simulink model "AD_Stepper_Simulation"  (Simulink 10.0)
settings: Solver=FixedStepDiscrete  StartTime=0.0  StopTime=10  FixedStep=Ts  RelTol=1e-3
InitFcn:
  | Ts = 0.01;      % model sample time
  | Tmax = 0.5;   % maximum time per "tick"
undefined symbols (not defined in the file): AD_Stepper_motor_lib, P_PulsGeber, P_WaveDrive
libraries: simulink x7
settings Model: Creator=Admin  LastModifiedBy=bhisma
settings ConfigSet: Description=rtmc9s12target_R2008a
settings DataIOCC: LimitDataPoints=on  SignalLoggingSaveFormat=ModelDataLogs  SaveOutput=off  SaveTime=off  SignalLoggingName=sigsOut
settings OptimizationCC: ExpressionDepthLimit=2147483647  InitFltsAndDblsToZero=on
settings DebuggingCC: SaveWithParameterizedLinksMsg=none  SignalResolutionControl=TryResolveAllWithWarning  MultiTaskDSMMsg=warning  MultiTaskCondExecSysMsg=none  FcnCallInpInsideContextMsg=warning  StateNameClashWarn=warning
settings HardwareCC: ProdBitPerInt=16  ProdBitPerPointer=16  ProdBitPerSizeT=16  ProdBitPerPtrDiffT=16  ProdEndianess=BigEndian  ProdWordSize=16  ProdHWDeviceType=Motorola HC12  TargetHWDeviceType=32-bit Generic  ProdEqTarget=off
settings RTWCC: GenerateMakefile=off
settings GRTTargetCC: TargetFcnLib=ansi_tfl_tmw.mat  GeneratePreprocessorConditionals=Disable all
settings ConfigComp: CovExternalEMLEnable=off

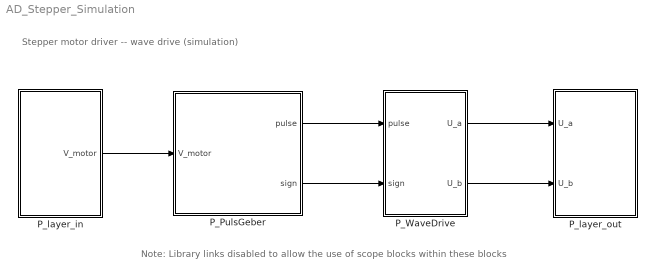
== system AD_Stepper_Simulation ==
  note: Stepper motor driver -- wave drive (simulation)
  note: Note: Library links disabled to allow the use of scope blocks within these blocks
  P_PulsGeber : Subsystem  AncestorBlock=AD_Stepper_motor_lib/P_PulsGeber  TreatAsAtomicUnit=on  SystemSampleTime=Ts
  P_WaveDrive : Subsystem  AncestorBlock=AD_Stepper_motor_lib/P_WaveDrive  TreatAsAtomicUnit=on  SystemSampleTime=Ts
  P_layer_in : Subsystem  TreatAsAtomicUnit=on
  P_layer_out : Subsystem  TreatAsAtomicUnit=on  SystemSampleTime=Ts
  wires:
  P_PulsGeber/1(pulse) -> P_WaveDrive/1(pulse)
  P_PulsGeber/2(sign) -> P_WaveDrive/2(sign)
  P_layer_in/1(V_motor) -> P_PulsGeber/1(V_motor)
  P_WaveDrive/1(U_a) -> P_layer_out/1(U_a)
  P_WaveDrive/2(U_b) -> P_layer_out/2(U_b)

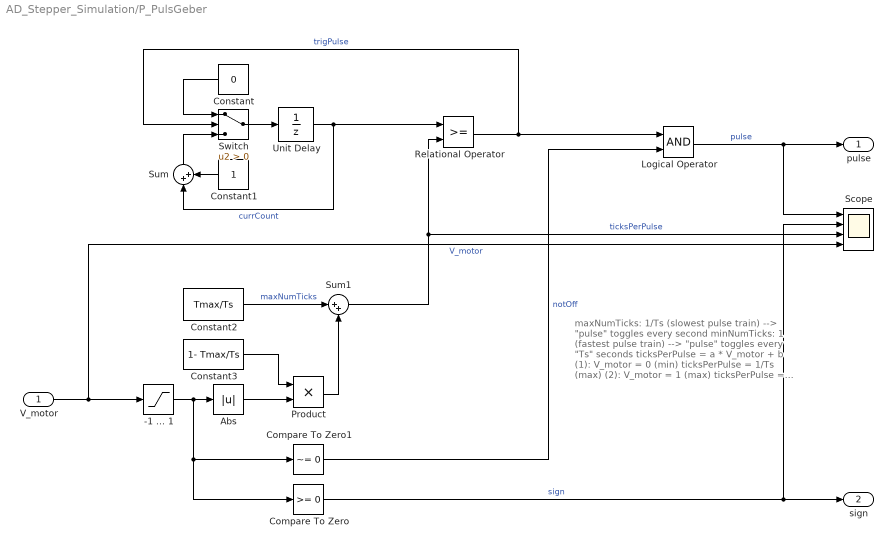
== system AD_Stepper_Simulation/P_PulsGeber ==
  note: maxNumTicks:  1/Ts   (slowest pulse train)
      | --> "pulse" toggles every second
      | minNumTicks: 1  (fastest pulse train)
      | --> "pulse" toggles every "Ts" seconds
      |
      | ticksPerPulse = a * V_motor + b
      |
      | (1):  V_motor = 0 (min)
      |        ticksPerPulse = 1/Ts (max)
      | (2):  V_motor = 1 (max)
      |        ticksPerPulse = 1 (min)
      |
      | (1):  1/Ts = b
      | (2):  1 = a * 1 + b   <=>   a = 1 - 1/Ts
      |
      | ticksPerPulse = (1 - 1/Ts) * V_motor + 1/Ts
  V_motor : Inport
  -1 ... 1 : Saturate  UpperLimit=1  LowerLimit=-1
  Abs : Abs
  Compare To Zero : simulink/Logic and Bit Operations/Compare To Zero  SystemSampleTime=-1  relop=>=  LogicOutDataTypeMode=boolean  ZeroCross=off
  Compare To Zero1 : simulink/Logic and Bit Operations/Compare To Zero  SystemSampleTime=-1  relop=~=  LogicOutDataTypeMode=boolean  ZeroCross=off
  Constant : Constant  Value=0
  Constant1 : Constant
  Constant2 : Constant  Value=Tmax/Ts
  Constant3 : Constant  Value=1- Tmax/Ts
  Logical Operator : Logic  AllPortsSameDT=off  OutDataTypeStr=boolean
  Product : Product  RndMeth=Zero
  Relational Operator : RelationalOperator  OutDataTypeStr=boolean  RndMeth=Nearest
  Scope : Scope  NumInputPorts=4
  Sum : Sum  Inputs=|++
  Sum1 : Sum  Inputs=|++
  Switch : Switch  Criteria=u2 > Threshold
  Unit Delay : UnitDelay  SampleTime=Ts
  pulse : Outport
  sign : Outport  Port=2
  wires:
  Compare To Zero1/1 -> Logical Operator/2  "notOff"
  Logical Operator/1 -> Scope/1, pulse/1  "pulse"
  V_motor/1 -> Scope/4, -1 ... 1/1  "V_motor"
  Sum1/1 -> Scope/3, Relational Operator/2  "ticksPerPulse"
  -1 ... 1/1 -> Compare To Zero1/1, Compare To Zero/1, Abs/1
  Constant3/1 -> Product/1
  Abs/1 -> Product/2
  Constant1/1 -> Sum/2
  Sum/1 -> Switch/3
  Switch/1 -> Unit Delay/1
  Unit Delay/1 -> Sum/1, Relational Operator/1  "currCount"
  Relational Operator/1 -> Logical Operator/1, Switch/2  "trigPulse"
  Constant/1 -> Switch/1
  Compare To Zero/1 -> Scope/2, sign/1  "sign"
  Product/1 -> Sum1/2
  Constant2/1 -> Sum1/1  "maxNumTicks"

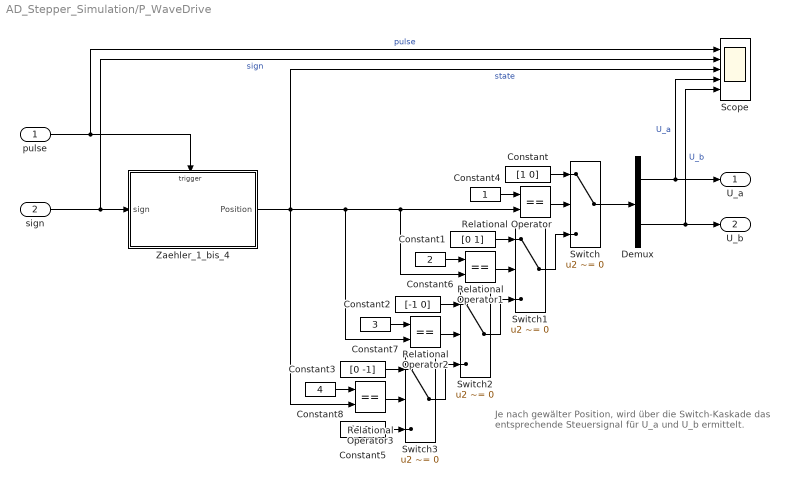
== system AD_Stepper_Simulation/P_WaveDrive ==
  note: Je nach gewälter Position, wird über die Switch-Kaskade
      | das entsprechende Steuersignal für U_a und U_b
      | ermittelt.
  pulse : Inport
  sign : Inport  Port=2
  Constant : Constant  Value=[1 0]
  Constant1 : Constant  Value=[0 1]
  Constant2 : Constant  Value=[-1 0]
  Constant3 : Constant  Value=[0 -1]
  Constant4 : Constant
  Constant5 : Constant  Value=[0 0]
  Constant6 : Constant  Value=2
  Constant7 : Constant  Value=3
  Constant8 : Constant  Value=4
  Demux : Demux  Outputs=2
  Relational Operator{,1..3} (4 alike) : RelationalOperator  Operator===  OutDataTypeStr=boolean  RndMeth=Nearest
  Scope : Scope  NumInputPorts=5
  Switch{,1..3} (4 alike) : Switch  Criteria=u2 ~= 0
  Zaehler_1_bis_4 : Subsystem  TreatAsAtomicUnit=on
  U_a : Outport
  U_b : Outport  Port=2
  wires:
  Constant4/1 -> Relational Operator/1
  Constant/1 -> Switch/1
  Relational Operator/1 -> Switch/2
  Constant6/1 -> Relational Operator1/1
  Constant1/1 -> Switch1/1
  Relational Operator1/1 -> Switch1/2
  Switch1/1 -> Switch/3
  Constant7/1 -> Relational Operator2/1
  Constant2/1 -> Switch2/1
  Relational Operator2/1 -> Switch2/2
  Switch2/1 -> Switch1/3
  Constant8/1 -> Relational Operator3/1
  Constant3/1 -> Switch3/1
  Relational Operator3/1 -> Switch3/2
  Switch3/1 -> Switch2/3
  Constant5/1 -> Switch3/3
  Switch/1 -> Demux/1
  pulse/1 -> Scope/1, Zaehler_1_bis_4/Trigger  "pulse"
  sign/1 -> Scope/2, Zaehler_1_bis_4/1(sign)  "sign"
  Zaehler_1_bis_4/1(Position) -> Relational Operator/2, Relational Operator1/2, Relational Operator2/2, Relational Operator3/2, Scope/3  "state"
  Demux/1 -> Scope/4, U_a/1  "U_a"
  Demux/2 -> Scope/5, U_b/1  "U_b"

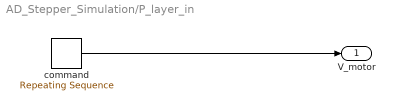
== system AD_Stepper_Simulation/P_layer_in ==
  command : simulink/Sources/Repeating Sequence  SystemSampleTime=-1  rep_seq_t=[0:10]  rep_seq_y=[0 0 -0.8 -0.8 0 0 0.5 0.9 0.8 0.2 0]
  V_motor : Outport
  wires:
  command/1 -> V_motor/1

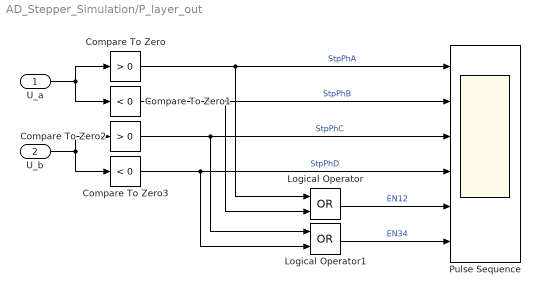
== system AD_Stepper_Simulation/P_layer_out ==
  U_a : Inport
  U_b : Inport  Port=2
  Compare To Zero : simulink/Logic and Bit Operations/Compare To Zero  SystemSampleTime=-1  relop=>  LogicOutDataTypeMode=boolean  ZeroCross=off
  Compare To Zero1 : simulink/Logic and Bit Operations/Compare To Zero  SystemSampleTime=-1  relop=<  LogicOutDataTypeMode=boolean  ZeroCross=off
  Compare To Zero2 : simulink/Logic and Bit Operations/Compare To Zero  SystemSampleTime=-1  relop=>  LogicOutDataTypeMode=boolean  ZeroCross=off
  Compare To Zero3 : simulink/Logic and Bit Operations/Compare To Zero  SystemSampleTime=-1  relop=<  LogicOutDataTypeMode=boolean  ZeroCross=off
  Logical Operator : Logic  Operator=OR  AllPortsSameDT=off  OutDataTypeStr=boolean
  Logical Operator1 : Logic  Operator=OR  AllPortsSameDT=off  OutDataTypeStr=boolean
  Pulse Sequence : Scope  NumInputPorts=6
  wires:
  U_a/1 -> Compare To Zero/1, Compare To Zero1/1
  U_b/1 -> Compare To Zero3/1, Compare To Zero2/1
  Compare To Zero/1 -> Logical Operator/1, Pulse Sequence/1  "StpPhA"
  Compare To Zero1/1 -> Logical Operator/2, Pulse Sequence/2  "StpPhB"
  Compare To Zero2/1 -> Logical Operator1/1, Pulse Sequence/3  "StpPhC"
  Compare To Zero3/1 -> Logical Operator1/2, Pulse Sequence/4  "StpPhD"
  Logical Operator/1 -> Pulse Sequence/5  "EN12"
  Logical Operator1/1 -> Pulse Sequence/6  "EN34"

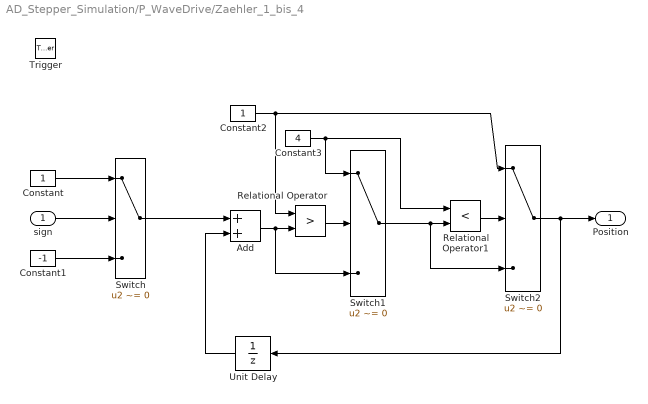
== system AD_Stepper_Simulation/P_WaveDrive/Zaehler_1_bis_4 ==
  sign : Inport
  Trigger : TriggerPort  VariantControl=(inherit)
  Add : Sum
  Constant : Constant
  Constant1 : Constant  Value=-1
  Constant2 : Constant
  Constant3 : Constant  Value=4
  Relational Operator : RelationalOperator  Operator=>  OutDataTypeStr=boolean  RndMeth=Nearest
  Relational Operator1 : RelationalOperator  Operator=<  OutDataTypeStr=boolean  RndMeth=Nearest
  Switch : Switch  Criteria=u2 ~= 0
  Switch1 : Switch  Criteria=u2 ~= 0
  Switch2 : Switch  Criteria=u2 ~= 0
  Unit Delay : UnitDelay  InitialCondition=1  SampleTime=-1
  Position : Outport
  wires:
  Constant/1 -> Switch/1
  sign/1 -> Switch/2
  Constant1/1 -> Switch/3
  Switch/1 -> Add/1
  Unit Delay/1 -> Add/2
  Constant2/1 -> Relational Operator/1, Switch2/1
  Add/1 -> Relational Operator/2, Switch1/3
  Constant3/1 -> Switch1/1, Relational Operator1/1
  Relational Operator/1 -> Switch1/2
  Switch1/1 -> Relational Operator1/2, Switch2/3
  Relational Operator1/1 -> Switch2/2
  Switch2/1 -> Position/1, Unit Delay/1
